simulink model "mat_acc"  (Simulink 8.7)
settings: Solver=VariableStepDiscrete  StartTime=0.0  StopTime=Accelerator_A10_param.endTime  MaxStep=1  RelTol=1e-3
PreLoadFcn:
  | % Run the setup script when the model is opened
  | setup_mat_acc;
InitFcn:
  | % Run the setup script again just before the
  | % model is run, so that any updates made
  | % after opening are applied.
  | setup_mat_acc;
undefined symbols (not defined in the file or in its folder): AdvDSPBChannelOutDisplay, dpoly, dspba_ChannelInVis, dspba_ChannelOutVis, dspba_internal_get_channel_ports, evalAionMaskParam, latency, primtype, value
libraries: DSPBAPrim x1114, DSPBAAvalonST x8, DSPBABase x5, DSPBAControl x2
(part 1 of 5)
Description:
  | DSP Builder Advanced Template for Template Design implementing Primitive Subsystems
settings Model: Creator=mjervis  LastModifiedBy=5g
settings DataIOCC: SignalLoggingSaveFormat=ModelDataLogs
settings OptimizationCC: ExpressionDepthLimit=2147483647
settings DebuggingCC: SolverPrmCheckMsg=warning  InheritedTsInSrcMsg=none  IntegerOverflowMsg=none  FcnCallInpInsideContextMsg=UseLocalSettings  AllowSymbolicDim=off  StateNameClashWarn=warning  IntegerSaturationMsg=none
settings GRTTargetCC: CombineOutputUpdateFcns=off  GRTInterface=on

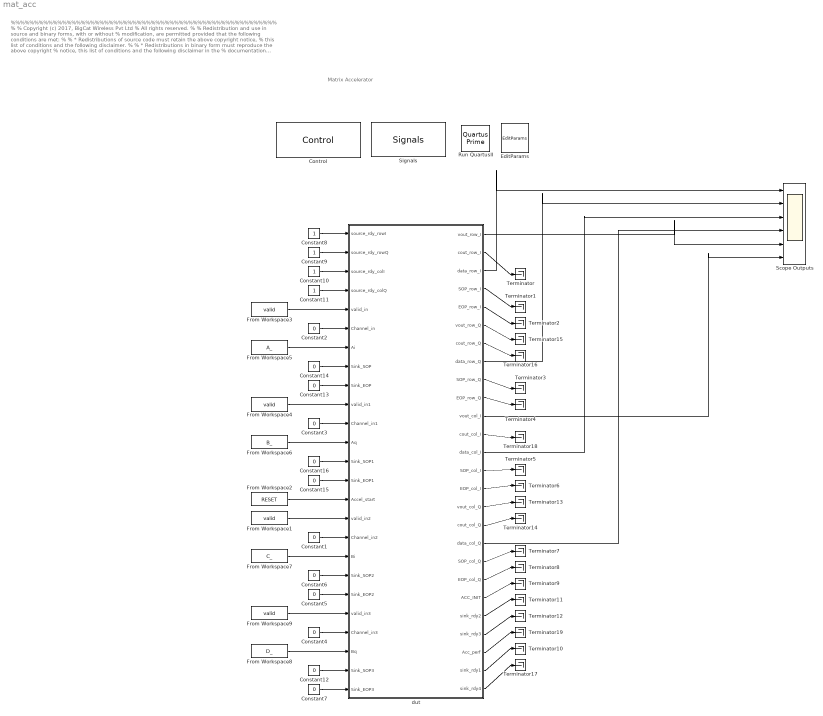
== system mat_acc ==
  note: %%%%%%%%%%%%%%%%%%%%%%%%%%%%%%%%%%%%%%%%%%%%%%%%%%%%%%%%%
      |  %
      |  % Copyright (c) 2017, BigCat Wireless Pvt Ltd
      |  % All rights reserved.
      |  %
      |  % Redistribution and use in source and binary forms, with or without
      |  % modification, are permitted provided that the following conditions are met:
      |  %
      |  %     * Redistributions of source code must retain the above copyright notice,
      |  %       this list of conditions and the following disclaimer.
      |  %
      |  %     * Redistributions in binary form must reproduce the above copyright
      |  %       notice, this list of conditions and the following disclaimer in the
      |  %       documentation and/or other materials provided with the distribution.
      |  %
      |  %     * Neither the name of the copyright holder nor the names of its contributors
      |  %       may be used to endorse or promote products derived from this software
      |  %       without specific prior written permission.
      |  %
      |  %
      |  %
      |  % THIS SOFTWARE IS PROVIDED BY THE COPYRIGHT HOLDERS AND CONTRIBUTORS "AS IS"
      |  % AND ANY EXPRESS OR IMPLIED WARRANTIES, INCLUDING, BUT NOT LIMITED TO, THE
      |  % IMPLIED WARRANTIES OF MERCHANTABILITY AND FITNESS FOR A PARTICULAR PURPOSE ARE
      |  % DISCLAIMED. IN NO EVENT SHALL THE COPYRIGHT HOLDER OR CONTRIBUTORS BE LIABLE
      |  % FOR ANY DIRECT, INDIRECT, INCIDENTAL, SPECIAL, EXEMPLARY, OR CONSEQUENTIAL
      |  % DAMAGES (INCLUDING, BUT NOT LIMITED TO, PROCUREMENT OF SUBSTITUTE GOODS OR
      |  % SERVICES; LOSS OF USE, DATA, OR PROFITS; OR BUSINESS INTERRUPTION) HOWEVER
      |  % CAUSED AND ON ANY THEORY OF LIABILITY, WHETHER IN CONTRACT, STRICT LIABILITY,
      |  % OR TORT (INCLUDING NEGLIGENCE OR OTHERWISE) ARISING IN ANY WAY OUT OF THE USE
      |  % OF THIS SOFTWARE, EVEN IF ADVISED OF THE POSSIBILITY OF SUCH DAMAGE.
      |  %
      |   %%%%%%%%%%%%%%%%%%%%%%%%%%%%%%%%%%%%%%%%%%%%%%%%%%%%%%%%%%
  note: Matrix Accelerator
  Constant{1..4} (4 alike) : Constant  Value=0  OutDataTypeStr=uint8
  Constant{8..11} (4 alike) : Constant  OutDataTypeStr=boolean
  Constant{5..7,12..16} (8 alike) : Constant  Value=0  OutDataTypeStr=boolean
  Control : DSPBABase/Control  generate=on  language=VHDL  destination=./rtl  destination_gui=./rtl  make_full_path=off  path_is_relative=on  autotestbench=on  signaldepth=2  coveragetestbench=off  logs=off  spacewidth=2  spacenum=1  addrwidth=10  datawidth=16  dataendian=Big Endian  hierarchicalnames=off  ramThresholdBits=-1  distRamThresholdBits=-1  mlabThresholdBits=-1  hardMultiplierThresholdLuts=-1  version=20090407  errorOnChanMismatch=1  errorOnGPIOMismatch=0  importModelsimResults=0  cycleAccurate=off  reinterpretCastMult=off  paramFile=mat_acc_params.xml
  EditParams : DSPBABase/EditParams  version=20090407
  From Workspace{1,3..4,9} (4 alike) : FromWorkspace  VariableName=valid  OutDataTypeStr=boolean  SampleTime=0
  From Workspace2 : FromWorkspace  VariableName=RESET  OutDataTypeStr=boolean  SampleTime=0
  From Workspace5 : FromWorkspace  VariableName=A_  SampleTime=0
  From Workspace6 : FromWorkspace  VariableName=B_  SampleTime=0
  From Workspace7 : FromWorkspace  VariableName=C_  SampleTime=0
  From Workspace8 : FromWorkspace  VariableName=D_  SampleTime=0
  "Run QuartusII " : DSPBABase/Quartus Prime  version=20090407
  Scope Outputs : Scope  NumInputPorts=6
  Signals : DSPBABase/Signals  clk=clk  freq=Accelerator_A10_param.ClockRate  margin=Accelerator_A10_param.ClockMargin  rst=areset  rstactive=High  bus=bus  enbusclock=off  busfreq=491.52  bussync=off  version=20090407
  Terminator{,1..19} (20 alike) : Terminator
  dut : Subsystem
  wires:
  Constant8/1 -> dut/1(source_rdy_rowI)
  Constant11/1 -> dut/4(source_rdy_colQ)
  Constant9/1 -> dut/2(source_rdy_rowQ)
  From Workspace2/1 -> dut/15(Accel_start)
  Constant10/1 -> dut/3(source_rdy_colI)
  Constant2/1 -> dut/6(Channel_in)
  Constant3/1 -> dut/11(Channel_in1)
  Constant14/1 -> dut/8(Sink_SOP)
  Constant13/1 -> dut/9(Sink_EOP)
  Constant16/1 -> dut/13(Sink_SOP1)
  Constant15/1 -> dut/14(Sink_EOP1)
  From Workspace3/1 -> dut/5(valid_in)
  From Workspace4/1 -> dut/10(valid_in1)
  dut/3(data_row_I) -> Scope Outputs/1
  dut/8(data_row_Q) -> Scope Outputs/2
  dut/13(data_col_I) -> Scope Outputs/3
  dut/18(data_col_Q) -> Scope Outputs/4
  dut/1(vout_row_I) -> Scope Outputs/5
  dut/11(vout_col_I) -> Scope Outputs/6
  dut/2(cout_row_I) -> Terminator/1
  dut/4(SOP_row_I) -> Terminator1/1
  dut/5(EOP_row_I) -> Terminator2/1
  dut/9(SOP_row_Q) -> Terminator3/1
  dut/10(EOP_row_Q) -> Terminator4/1
  dut/14(SOP_col_I) -> Terminator5/1
  dut/15(EOP_col_I) -> Terminator6/1
  dut/19(SOP_col_Q) -> Terminator7/1
  dut/20(EOP_col_Q) -> Terminator8/1
  dut/21(ACC_INIT) -> Terminator9/1
  dut/22(sink_rdy2) -> Terminator11/1
  dut/23(sink_rdy3) -> Terminator12/1
  dut/16(vout_col_Q) -> Terminator13/1
  dut/17(cout_col_Q) -> Terminator14/1
  dut/6(vout_row_Q) -> Terminator15/1
  dut/7(cout_row_Q) -> Terminator16/1
  dut/12(cout_col_I) -> Terminator18/1
  dut/24(Acc_perf) -> Terminator19/1
  From Workspace5/1 -> dut/7(Ai)
  From Workspace6/1 -> dut/12(Aq)
  From Workspace7/1 -> dut/18(Bi)
  From Workspace8/1 -> dut/23(Bq)
  From Workspace1/1 -> dut/16(valid_in2)
  From Workspace9/1 -> dut/21(valid_in3)
  Constant1/1 -> dut/17(Channel_in2)
  Constant4/1 -> dut/22(Channel_in3)
  Constant6/1 -> dut/19(Sink_SOP2)
  Constant5/1 -> dut/20(Sink_EOP2)
  Constant12/1 -> dut/24(Sink_SOP3)
  Constant7/1 -> dut/25(Sink_EOP3)
  dut/26(sink_rdy4) -> Terminator17/1
  dut/25(sink_rdy1) -> Terminator10/1

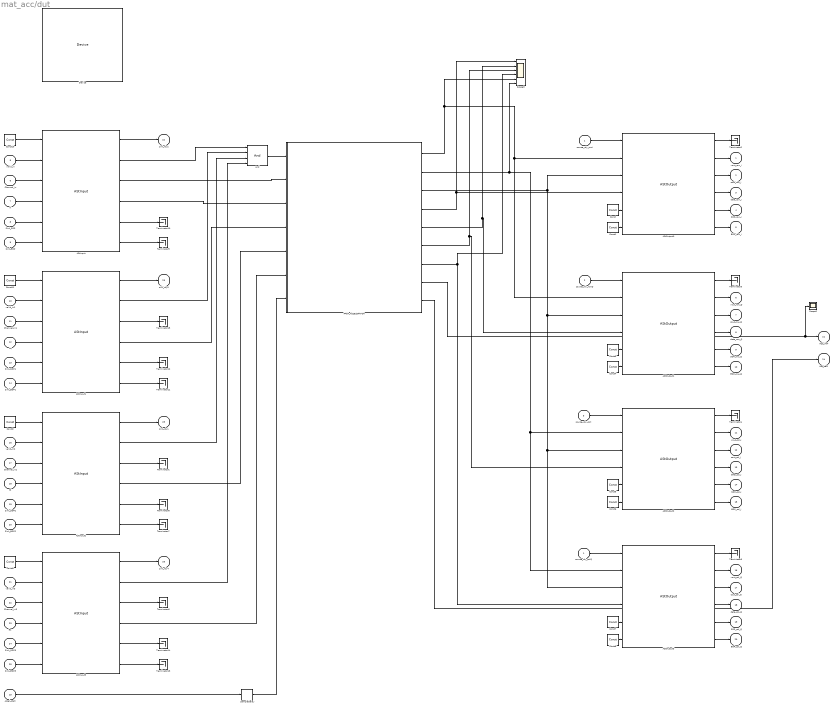
== system mat_acc/dut ==
  source_rdy_rowI : Inport
  source_rdy_rowQ : Inport  Port=2
  source_rdy_colI : Inport  Port=3
  source_rdy_colQ : Inport  Port=4
  valid_in : Inport  Port=5
  Channel_in : Inport  Port=6
  Ai : Inport  Port=7
  Sink_SOP : Inport  Port=8
  Sink_EOP : Inport  Port=9
  valid_in1 : Inport  Port=10
  Channel_in1 : Inport  Port=11
  Aq : Inport  Port=12
  Sink_SOP1 : Inport  Port=13
  Sink_EOP1 : Inport  Port=14
  Accel_start : Inport  Port=15
  valid_in2 : Inport  Port=16
  Channel_in2 : Inport  Port=17
  Bi : Inport  Port=18
  Sink_SOP2 : Inport  Port=19
  Sink_EOP2 : Inport  Port=20
  valid_in3 : Inport  Port=21
  Channel_in3 : Inport  Port=22
  Bq : Inport  Port=23
  Sink_SOP3 : Inport  Port=24
  Sink_EOP3 : Inport  Port=25
  AStInput : DSPBAAvalonST/AStInput
      link override ChannelOut: value=3  packetBeginEnabled=off  latency=0
  AStInput1 : DSPBAAvalonST/AStInput
      link override ChannelOut: value=3  packetBeginEnabled=off  latency=0
  AStInput2 : DSPBAAvalonST/AStInput
      link override ChannelOut: value=3  packetBeginEnabled=off  latency=0
  AStInput3 : DSPBAAvalonST/AStInput
      link override ChannelOut: value=3  packetBeginEnabled=off  latency=0
  AStOutput0 : DSPBAAvalonST/AStOutput  fifo_setup=[32 1 20]
      link override ChannelOut: value=4  packetBeginEnabled=off  latency=0
  AStOutput1 : DSPBAAvalonST/AStOutput  fifo_setup=[32 1 20]
      link override ChannelOut: value=4  packetBeginEnabled=off  latency=0
  AStOutput2 : DSPBAAvalonST/AStOutput  fifo_setup=[32 1 20]
      link override ChannelOut: value=4  packetBeginEnabled=off  latency=0
  AStOutput3 : DSPBAAvalonST/AStOutput  fifo_setup=[32 1 20]
      link override ChannelOut: value=4  packetBeginEnabled=off  latency=0
  And : DSPBAPrim/And  primtype=and  nInputs=4  nOutputs=1  omode=Inherit via internal rule  otype=sfix(16)  scale=2^-15  rndmethod=Unbiased  factor=1  satmethod=Symmetric  shift_vec=[0 1 2 -1]  value=0  inPortNames=[' '; ' '; ' '; ' '; ' '; ' '; ' '; ' '; ' '; ' '; ' '; ' '; ' '; ' '; ' '; ' '; ]  outPortNames=[' ']  dspbaimage=dspba_prim.jpg  text=fprintf('&');  style=Optimised  visibilities=8+2  version=20090407
  Const{,1,3..8} (8 alike) : DSPBAPrim/Const  primtype=const  nInputs=0  nOutputs=1  omode=boolean  otype=sfix(16)  scale=2^-15  rndmethod=Unbiased  factor=1  satmethod=Symmetric  shift_vec=[0 1 2 -1]  value=0  inPortNames=['+'; '+';]  outPortNames=[' ']  dspbaimage=dspba_prim.jpg  text=fprintf('%s', num2str(value));  style=Optimised  visibilities=8 + 1024  floatPrecision=float32_m23  version=20120820
  Const{2,9..11} (4 alike) : DSPBAPrim/Const  primtype=const  nInputs=0  nOutputs=1  omode=boolean  otype=sfix(16)  scale=2^-15  rndmethod=Unbiased  factor=1  satmethod=Symmetric  shift_vec=[0 1 2 -1]  value=1  inPortNames=['+'; '+';]  outPortNames=[' ']  dspbaimage=dspba_prim.jpg  text=fprintf('%s', num2str(value));  style=Optimised  visibilities=8 + 1024  floatPrecision=float32_m23  version=20120820
  Device : DSPBABase/Device  family=Arria 10  deviceMember=Arria 10  stratix4device=Stratix IV E  hardcopy4device=HardCopy IV E  stratix5device=Stratix V GX  device=10AS066N3F40E2SGE2  speed=2  stratixSpeed=-5  stratix2Speed=-3  stratix3Speed=-2  stratix4gxSpeed=-2  stratix4gtSpeed=-1  cyclone2Speed=-6  cyclone3Speed=-7  arria2Speed=-4  cyclone4eSpeed=-8  stratix5Speed=-3  arria5Speed=-4  arriaSpeed=-6  cyclone3lsSpeed=-7  cyclone5Speed=-6  arria2gzSpeed=-3  nightFurySpeed=-2  ecp2Speed=-7  hardcopycompat=off  version=20140217  max10flashmode=off  max10nomeminit=off
  FPGA_ACCELERATOR : Subsystem
  SampleDelay : DSPBAPrim/SampleDelay  primtype=sampdelay  nInputs=1  nOutputs=1  omode=Inherit via internal rule  otype=sfix(16)  scale=2^-15  rndmethod=Unbiased  factor=1  satmethod=Symmetric  shift_vec=[0 1 2 -1]  value=1  inPortNames=[' '; ' ';]  outPortNames=[' ']  dspbaimage=dspba_prim.jpg  text=dpoly(1, eye(1,value+1), 'z')  style=Optimised  visibilities=8 + 1024 + 2^17 + 2^18  flexible=off  slackgroup=0  augmented=0  version=20090407  advOptions=[]
  Scope2 : Scope
  Scope3 : Scope  NumInputPorts=6
  Terminator{1..15} (15 alike) : Terminator
  vout_row_I : Outport
  cout_row_I : Outport  Port=2
  data_row_I : Outport  Port=3
  SOP_row_I : Outport  Port=4
  EOP_row_I : Outport  Port=5
  vout_row_Q : Outport  Port=6
  cout_row_Q : Outport  Port=7
  data_row_Q : Outport  Port=8
  SOP_row_Q : Outport  Port=9
  EOP_row_Q : Outport  Port=10
  vout_col_I : Outport  Port=11
  cout_col_I : Outport  Port=12
  data_col_I : Outport  Port=13
  SOP_col_I : Outport  Port=14
  EOP_col_I : Outport  Port=15
  vout_col_Q : Outport  Port=16
  cout_col_Q : Outport  Port=17
  data_col_Q : Outport  Port=18
  SOP_col_Q : Outport  Port=19
  EOP_col_Q : Outport  Port=20
  ACC_INIT : Outport  Port=21
  sink_rdy2 : Outport  Port=22
  sink_rdy3 : Outport  Port=23
  Acc_perf : Outport  Port=24
  sink_rdy1 : Outport  Port=25
  sink_rdy4 : Outport  Port=26
  wires:
  FPGA_ACCELERATOR/1(R_vout) -> AStOutput0/2, AStOutput1/2, Scope3/5
  FPGA_ACCELERATOR/3(cout) -> AStOutput1/3, AStOutput2/3, AStOutput3/3, AStOutput0/3
  FPGA_ACCELERATOR/4(Row_i) -> Scope3/1, AStOutput0/4
  AStOutput0/2 -> vout_row_I/1
  AStOutput0/3 -> cout_row_I/1
  source_rdy_rowI/1 -> AStOutput0/1
  AStOutput0/1 -> Terminator2/1
  Const/1 -> AStOutput0/5
  Const1/1 -> AStOutput0/6
  AStOutput0/4 -> data_row_I/1
  FPGA_ACCELERATOR/2(Col_vout) -> AStOutput2/2, AStOutput3/2, Scope3/6
  FPGA_ACCELERATOR/5(Row_q) -> Scope3/2, AStOutput1/4
  FPGA_ACCELERATOR/6(Col_i) -> Scope3/3, AStOutput2/4
  FPGA_ACCELERATOR/7(Col_q) -> Scope3/4, AStOutput3/4
  Const3/1 -> AStOutput1/5
  Const4/1 -> AStOutput1/6
  Const5/1 -> AStOutput2/5
  Const6/1 -> AStOutput2/6
  Const7/1 -> AStOutput3/5
  Const8/1 -> AStOutput3/6
  source_rdy_rowQ/1 -> AStOutput1/1
  source_rdy_colI/1 -> AStOutput2/1
  source_rdy_colQ/1 -> AStOutput3/1
  AStOutput3/1 -> Terminator5/1
  AStOutput2/1 -> Terminator4/1
  AStOutput1/1 -> Terminator3/1
  AStOutput1/2 -> vout_row_Q/1
  AStOutput1/3 -> cout_row_Q/1
  AStOutput1/4 -> data_row_Q/1
  AStOutput2/2 -> vout_col_I/1
  AStOutput2/3 -> cout_col_I/1
  AStOutput2/4 -> data_col_I/1
  AStOutput3/2 -> vout_col_Q/1
  AStOutput3/3 -> cout_col_Q/1
  AStOutput3/4 -> data_col_Q/1
  AStOutput0/5 -> SOP_row_I/1
  AStOutput0/6 -> EOP_row_I/1
  AStOutput1/5 -> SOP_row_Q/1
  AStOutput1/6 -> EOP_row_Q/1
  AStOutput3/5 -> SOP_col_Q/1
  AStOutput3/6 -> EOP_col_Q/1
  AStOutput2/5 -> SOP_col_I/1
  AStOutput2/6 -> EOP_col_I/1
  AStInput/5 -> Terminator10/1
  AStInput/6 -> Terminator9/1
  AStInput1/5 -> Terminator12/1
  AStInput1/6 -> Terminator11/1
  Channel_in/1 -> AStInput/3
  valid_in/1 -> AStInput/2
  Ai/1 -> AStInput/4
  Sink_SOP/1 -> AStInput/5
  Sink_EOP/1 -> AStInput/6
  Channel_in1/1 -> AStInput1/3
  valid_in1/1 -> AStInput1/2
  Aq/1 -> AStInput1/4
  Sink_SOP1/1 -> AStInput1/5
  Sink_EOP1/1 -> AStInput1/6
  And/1 -> FPGA_ACCELERATOR/1(Valid_in)
  AStInput/2 -> And/1
  AStInput1/2 -> And/2
  AStInput/1 -> sink_rdy2/1
  AStInput1/1 -> sink_rdy3/1
  AStInput/3 -> FPGA_ACCELERATOR/2(channel_in)
  AStInput1/3 -> Terminator15/1
  SampleDelay/1 -> FPGA_ACCELERATOR/7(Start_of_operation)
  Const10/1 -> AStInput/1
  Const11/1 -> AStInput1/1
  Accel_start/1 -> SampleDelay/1
  FPGA_ACCELERATOR/9(Acc_perf) -> Acc_perf/1
  FPGA_ACCELERATOR/8(Acc_init) -> Scope2/1, ACC_INIT/1
  AStInput/4 -> FPGA_ACCELERATOR/3(Ai)
  AStInput1/4 -> FPGA_ACCELERATOR/4(Aq)
  Channel_in2/1 -> AStInput2/3
  valid_in2/1 -> AStInput2/2
  Bi/1 -> AStInput2/4
  Sink_SOP2/1 -> AStInput2/5
  Sink_EOP2/1 -> AStInput2/6
  Const2/1 -> AStInput2/1
  Channel_in3/1 -> AStInput3/3
  valid_in3/1 -> AStInput3/2
  Bq/1 -> AStInput3/4
  Sink_SOP3/1 -> AStInput3/5
  Sink_EOP3/1 -> AStInput3/6
  Const9/1 -> AStInput3/1
  AStInput2/1 -> sink_rdy1/1
  AStInput3/1 -> sink_rdy4/1
  AStInput2/2 -> And/3
  AStInput3/2 -> And/4
  AStInput2/3 -> Terminator1/1
  AStInput3/3 -> Terminator6/1
  AStInput2/5 -> Terminator8/1
  AStInput2/6 -> Terminator7/1
  AStInput3/5 -> Terminator14/1
  AStInput3/6 -> Terminator13/1
  AStInput2/4 -> FPGA_ACCELERATOR/5(Bi)
  AStInput3/4 -> FPGA_ACCELERATOR/6(Bq)

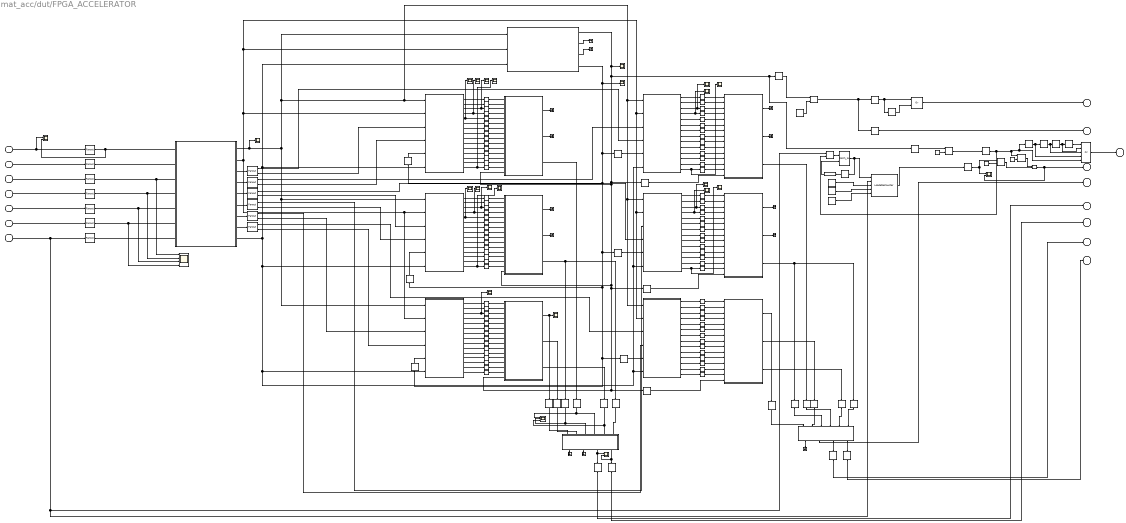
== system mat_acc/dut/FPGA_ACCELERATOR ==
  Valid_in : Inport
  channel_in : Inport  Port=2
  Ai : Inport  Port=3
  Aq : Inport  Port=4
  Bi : Inport  Port=5
  Bq : Inport  Port=6
  Start_of_operation : Inport  Port=7
  12FP_MAC : Subsystem
  12FP_MAC1 : Subsystem
  12FP_MAC2 : Subsystem
  12FP_MUX : Subsystem
  12FP_MUX1 : Subsystem
  12FP_MUX2 : Subsystem
  13FP_MAC : Subsystem
  13FP_MAC1 : Subsystem
  13FP_MAC2 : Subsystem
  13FP_MUX : Subsystem
  13FP_MUX1 : Subsystem
  13FP_MUX2 : Subsystem
  COLUMN_I_and_Q : Subsystem
  CmpEQ : DSPBAPrim/CmpEQ  primtype=cmpeq  nInputs=2  nOutputs=1  omode=boolean  otype=sfix(16)  scale=2^-15  rndmethod=Unbiased  factor=1  satmethod=Symmetric  shift_vec=[0 1 2 -1]  value=0  inPortNames=[' '; ' ';]  outPortNames=[' ']  dspbaimage=dspba_prim.jpg  text=fprintf('==');  style=Optimised  visibilities=0  advOptions=[]  version=20130117
  CmpGE : DSPBAPrim/CmpGE  primtype=cmpgte  nInputs=2  nOutputs=1  omode=boolean  otype=sfix(16)  scale=2^-15  rndmethod=Unbiased  factor=1  satmethod=Symmetric  shift_vec=[0 1 2 -1]  value=0  inPortNames=['a'; 'b';]  outPortNames=[' ']  dspbaimage=dspba_prim.jpg  text=fprintf('a>=b');  style=Optimised  visibilities=0  advOptions=[]  version=20130117
  Const : DSPBAPrim/Const  primtype=const  nInputs=0  nOutputs=1  omode=Inherit via internal rule  otype=sfix(16)  scale=2^-15  rndmethod=Unbiased  factor=1  satmethod=Symmetric  shift_vec=[0 1 2 -1]  value=1  inPortNames=['+'; '+';]  outPortNames=[' ']  dspbaimage=dspba_prim.jpg  text=fprintf('%s', num2str(value));  style=Optimised  visibilities=8 + 1024  floatPrecision=float32_m23  version=20120820
  Const1 : DSPBAPrim/Const  primtype=const  nInputs=0  nOutputs=1  omode=Inherit via internal rule  otype=sfix(16)  scale=2^-15  rndmethod=Unbiased  factor=1  satmethod=Symmetric  shift_vec=[0 1 2 -1]  value=1  inPortNames=['+'; '+';]  outPortNames=[' ']  dspbaimage=dspba_prim.jpg  text=fprintf('%s', num2str(value));  style=Optimised  visibilities=8 + 1024  floatPrecision=float32_m23  version=20120820
  Const2 : DSPBAPrim/Const  primtype=const  nInputs=0  nOutputs=1  omode=Inherit via internal rule  otype=sfix(16)  scale=2^-15  rndmethod=Unbiased  factor=1  satmethod=Symmetric  shift_vec=[0 1 2 -1]  value=0  inPortNames=['+'; '+';]  outPortNames=[' ']  dspbaimage=dspba_prim.jpg  text=fprintf('%s', num2str(value));  style=Optimised  visibilities=8 + 1024  floatPrecision=float32_m23  version=20120820
  Const3 : DSPBAPrim/Const  primtype=const  nInputs=0  nOutputs=1  omode=Inherit via internal rule  otype=sfix(16)  scale=2^-15  rndmethod=Unbiased  factor=1  satmethod=Symmetric  shift_vec=[0 1 2 -1]  value=100000  inPortNames=['+'; '+';]  outPortNames=[' ']  dspbaimage=dspba_prim.jpg  text=fprintf('%s', num2str(value));  style=Optimised  visibilities=8 + 1024  floatPrecision=float32_m23  version=20120820
  Const4 : DSPBAPrim/Const  primtype=const  nInputs=0  nOutputs=1  omode=Inherit via internal rule  otype=sfix(16)  scale=2^-15  rndmethod=Unbiased  factor=1  satmethod=Symmetric  shift_vec=[0 1 2 -1]  value=1  inPortNames=['+'; '+';]  outPortNames=[' ']  dspbaimage=dspba_prim.jpg  text=fprintf('%s', num2str(value));  style=Optimised  visibilities=8 + 1024  floatPrecision=float32_m23  version=20120820
  Const6 : DSPBAPrim/Const  primtype=const  nInputs=0  nOutputs=1  omode=boolean  otype=sfix(16)  scale=2^-15  rndmethod=Unbiased  factor=1  satmethod=Symmetric  shift_vec=[0 1 2 -1]  value=1  inPortNames=['+'; '+';]  outPortNames=[' ']  dspbaimage=dspba_prim.jpg  text=fprintf('%s', num2str(value));  style=Optimised  visibilities=8 + 1024  floatPrecision=float32_m23  version=20120820
  Const7 : DSPBAPrim/Const  primtype=const  nInputs=0  nOutputs=1  omode=Specify via dialog  otype=ufix(1)  scale=2^0  rndmethod=Unbiased  factor=1  satmethod=Symmetric  shift_vec=[0 1 2 -1]  value=1  inPortNames=['+'; '+';]  outPortNames=[' ']  dspbaimage=dspba_prim.jpg  text=fprintf('%s', num2str(value));  style=Optimised  visibilities=8 + 1024  floatPrecision=float32_m23  version=20120820
  Convert : DSPBAPrim/Convert  primtype=convert  nInputs=1  nOutputs=1  omode=boolean  otype=sfix(16)  scale=2^-15  rndmethod=Unbiased  factor=1  satmethod=None  shift_vec=[0 1 2 -1]  value=round([0:255]/17)  inPortNames=[' '; ' ';]  outPortNames=[' '; 'c']  dspbaimage=dspba_prim.jpg  text=fprintf('convert');  style=Optimised  visibilities=8+64+256+2^17  clipdetect=off  floatPrecision=float32_m23  advOptions=[]  version=20130211
  Counter_control_logic : Subsystem
  Fanout{,1..6,13..115} (110 alike) : DSPBAPrim/Fanout  primtype=fanout  nInputs=1  nOutputs=evalAionMaskParam(gcb,'value',1)  omode=Inherit via internal rule  otype=sfix(16)  scale=2^-15  rndmethod=Unbiased  factor=1  satmethod=Symmetric  shift_vec=[0 1 2 -1]  value=1  inPortNames=[' '; ' ';]  outPortNames=[' ']  dspbaimage=dspba_prim.jpg  text=fprintf('fanout')  style=Optimised  visibilities=2^10+2^18  version=20150501  uninit=off
  Fanout{7..12} (6 alike) : DSPBAPrim/Fanout  primtype=fanout  nInputs=1  nOutputs=evalAionMaskParam(gcb,'value',1)  omode=Inherit via internal rule  otype=sfix(16)  scale=2^-15  rndmethod=Unbiased  factor=1  satmethod=Symmetric  shift_vec=[0 1 2 -1]  value=2  inPortNames=[' '; ' ';]  outPortNames=[' ']  dspbaimage=dspba_prim.jpg  text=fprintf('fanout')  style=Optimised  visibilities=2^10+2^18  version=20150501  uninit=off
  Input_operations : Subsystem
  LShift : DSPBAPrim/LShift  primtype=lshift  nInputs=2  nOutputs=1  omode=Specify via dialog  otype=ufix(32)  scale=2^0  rndmethod=Unbiased  factor=1  satmethod=Symmetric  shift_vec=[0 1 2 -1]  value=0  inPortNames=['a'; 'b';]  outPortNames=[' ']  dspbaimage=dspba_prim.jpg  text=fprintf('a << b');  style=Optimised  visibilities=8  version=20090407
  LoadableCounter : DSPBAPrim/LoadableCounter  primtype=loadablecounter  nInputs=5  nOutputs=1  omode=Inherit via internal rule  otype=ufix(16)  scale=2^-0  rndmethod=Unbiased  factor=1  satmethod=Symmetric  shift_vec=[0 1 2 -1]  value=[0 1 0]  inPortNames=['en';'ld';'i ';'s ';'m ']  outPortNames=[' ']  dspbaimage=dspba_prim.jpg  text=fprintf('loadable\ncounter\n[%d %d %d]', value(1), value(2), value(3));  style=Optimised  visibilities=8 + 1024  version=20090407
  Not1 : DSPBAPrim/Not  primtype=not  nInputs=1  nOutputs=1  omode=Inherit via internal rule  otype=sfix(16)  scale=2^-15  rndmethod=Unbiased  factor=1  satmethod=Symmetric  shift_vec=[0 1 2 -1]  value=0  inPortNames=[' '; ' ';]  outPortNames=[' ']  dspbaimage=dspba_prim.jpg  text=fprintf('~');  style=Optimised  visibilities=8  version=20090407
  Or : DSPBAPrim/Or  primtype=or  nInputs=2  nOutputs=1  omode=Inherit via internal rule  otype=sfix(16)  scale=2^-15  rndmethod=Unbiased  factor=1  satmethod=Symmetric  shift_vec=[0 1 2 -1]  value=0  inPortNames=[' '; ' '; ' '; ' '; ' '; ' '; ' '; ' '; ' '; ' '; ' '; ' '; ' '; ' '; ' '; ' '; ]  outPortNames=[' ']  dspbaimage=dspba_prim.jpg  text=fprintf('|');  style=Optimised  visibilities=8+2  version=20090407
  Or1 : DSPBAPrim/Or  primtype=or  nInputs=2  nOutputs=1  omode=Inherit via internal rule  otype=sfix(16)  scale=2^-15  rndmethod=Unbiased  factor=1  satmethod=Symmetric  shift_vec=[0 1 2 -1]  value=0  inPortNames=[' '; ' '; ' '; ' '; ' '; ' '; ' '; ' '; ' '; ' '; ' '; ' '; ' '; ' '; ' '; ' '; ]  outPortNames=[' ']  dspbaimage=dspba_prim.jpg  text=fprintf('|');  style=Optimised  visibilities=8+2  version=20090407
  Or2 : DSPBAPrim/Or  primtype=or  nInputs=2  nOutputs=1  omode=Inherit via internal rule  otype=sfix(16)  scale=2^-15  rndmethod=Unbiased  factor=1  satmethod=Symmetric  shift_vec=[0 1 2 -1]  value=0  inPortNames=[' '; ' '; ' '; ' '; ' '; ' '; ' '; ' '; ' '; ' '; ' '; ' '; ' '; ' '; ' '; ' '; ]  outPortNames=[' ']  dspbaimage=dspba_prim.jpg  text=fprintf('|');  style=Optimised  visibilities=8+2  version=20090407
  Or3 : DSPBAPrim/Or  primtype=or  nInputs=5  nOutputs=1  omode=Inherit via internal rule  otype=sfix(16)  scale=2^-15  rndmethod=Unbiased  factor=1  satmethod=Symmetric  shift_vec=[0 1 2 -1]  value=0  inPortNames=[' '; ' '; ' '; ' '; ' '; ' '; ' '; ' '; ' '; ' '; ' '; ' '; ' '; ' '; ' '; ' '; ]  outPortNames=[' ']  dspbaimage=dspba_prim.jpg  text=fprintf('|');  style=Optimised  visibilities=8+2  version=20090407
  ROW_I_and_Q : Subsystem
  SampleDelay{3..5,93,95..96,98..99,105..108,110..115} (18 alike) : DSPBAPrim/SampleDelay  primtype=sampdelay  nInputs=1  nOutputs=1  omode=Inherit via internal rule  otype=sfix(16)  scale=2^-15  rndmethod=Unbiased  factor=1  satmethod=Symmetric  shift_vec=[0 1 2 -1]  value=1  inPortNames=[' '; ' ';]  outPortNames=[' ']  dspbaimage=dspba_prim.jpg  text=dpoly(1, eye(1,value+1), 'z')  style=Optimised  visibilities=8 + 1024 + 2^17 + 2^18  flexible=off  slackgroup=0  augmented=0  version=20090407  advOptions=[]
  SampleDelay109 : DSPBAPrim/SampleDelay  primtype=sampdelay  nInputs=1  nOutputs=1  omode=Inherit via internal rule  otype=sfix(16)  scale=2^-15  rndmethod=Unbiased  factor=1  satmethod=Symmetric  shift_vec=[0 1 2 -1]  value=8  inPortNames=[' '; ' ';]  outPortNames=[' ']  dspbaimage=dspba_prim.jpg  text=dpoly(1, eye(1,value+1), 'z')  style=Optimised  visibilities=8 + 1024 + 2^17 + 2^18  flexible=off  slackgroup=0  augmented=0  version=20090407  advOptions=[]
  SampleDelay94 : DSPBAPrim/SampleDelay  primtype=sampdelay  nInputs=1  nOutputs=1  omode=Inherit via internal rule  otype=sfix(16)  scale=2^-15  rndmethod=Unbiased  factor=1  satmethod=Symmetric  shift_vec=[0 1 2 -1]  value=11  inPortNames=[' '; ' ';]  outPortNames=[' ']  dspbaimage=dspba_prim.jpg  text=dpoly(1, eye(1,value+1), 'z')  style=Optimised  visibilities=8 + 1024 + 2^17 + 2^18  flexible=off  slackgroup=0  augmented=0  version=20090407  advOptions=[]
  Scope{,2,4..6,8..18,20..22} (19 alike) : Scope
  Scope1 : Scope  NumInputPorts=2
  Scope19 : Scope  NumInputPorts=2
  Scope23 : Scope  NumInputPorts=2
  Scope3 : Scope  NumInputPorts=3
  Scope7 : Scope  NumInputPorts=4
  Terminator{,1..4,7..9,11..15} (13 alike) : Terminator
  latch_1L : DSPBAControl/latch_1L
  latch_1L1 : DSPBAControl/latch_1L
  R_vout : Outport
  Col_vout : Outport  Port=2
  cout : Outport  Port=3
  Row_i : Outport  Port=4
  Row_q : Outport  Port=5
  Col_i : Outport  Port=6
  Col_q : Outport  Port=7
  Acc_init : Outport  Port=8
  Acc_perf : Outport  Port=9
  wires:
  Counter_control_logic/1(Count) -> SampleDelay4/1, 13FP_MUX2/16(MUX_select), SampleDelay5/1, 13FP_MUX1/16(MUX_select), 13FP_MUX/16(MUX_select), SampleDelay3/1, SampleDelay109/1, SampleDelay94/1, Scope/1
  Fanout9/1 -> 12FP_MAC1/4(Ai-Aq)
  13FP_MUX1/3((Ai-Aq)*Bq) -> Fanout104/1, Fanout102/1
  12FP_MUX2/3((Bi+Bq)*Aq) -> Fanout110/1
  13FP_MUX2/3(Aq*(Bi+Bq)) -> Fanout105/1
  12FP_MAC1/4(M1) -> Fanout75/1, Scope18/1
  12FP_MAC2/12(M9) -> Fanout97/1
  12FP_MAC1/12(M9) -> Fanout83/1
  12FP_MAC2/4(M1) -> Fanout89/1
  12FP_MAC2/7(M4) -> Fanout92/1
  12FP_MAC2/9(M6) -> Fanout94/1
  12FP_MAC1/3(M0) -> Fanout74/1, Scope6/1
  12FP_MAC2/1(vout) -> Fanout86/1
  12FP_MAC2/3(M0) -> Fanout88/1
  12FP_MUX/3((Bi-Bq)*Ai) -> Fanout109/1
  12FP_MAC/4(M1) -> Fanout61/1, Scope17/1
  12FP_MAC/6(M3) -> Fanout63/1
  12FP_MAC/10(M7) -> Fanout67/1
  12FP_MAC2/14(M11) -> Fanout99/1
  12FP_MAC1/13(M10) -> Fanout84/1
  12FP_MAC1/6(M3) -> Fanout77/1
  12FP_MAC1/7(M4) -> Fanout78/1
  12FP_MUX1/3(Bq*(Ai-Aq)) -> Fanout111/1, Fanout108/1
  12FP_MAC/13(M10) -> Fanout70/1
  12FP_MAC1/8(M5) -> Fanout79/1
  12FP_MAC2/8(M5) -> Fanout93/1
  12FP_MAC2/13(M10) -> Fanout98/1
  12FP_MAC2/11(M8) -> Fanout96/1
  12FP_MAC1/9(M6) -> Fanout80/1
  12FP_MAC1/2(cout) -> Fanout73/1
  12FP_MAC1/11(M8) -> Fanout82/1
  12FP_MAC1/10(M7) -> Fanout81/1
  12FP_MAC2/10(M7) -> Fanout95/1
  12FP_MAC2/5(M2) -> Fanout90/1
  12FP_MAC1/14(M11) -> Fanout85/1, Scope15/1
  12FP_MAC/11(M8) -> Fanout68/1
  12FP_MAC2/2(cout) -> Fanout87/1
  12FP_MAC/9(M6) -> Fanout66/1
  13FP_MAC1/6(M3) -> Fanout33/1
  13FP_MAC/4(M1) -> Fanout16/1, Scope9/1
  13FP_MAC2/10(M7) -> Fanout52/1
  13FP_MAC1/4(M1) -> Fanout31/1, Scope10/1
  13FP_MAC/9(M6) -> Fanout21/1
  12FP_MAC/8(M5) -> Fanout65/1
  13FP_MAC1/5(M2) -> Fanout32/1, Scope12/1
  12FP_MAC2/6(M3) -> Fanout91/1
  13FP_MAC/5(M2) -> Fanout17/1, Scope11/1
  13FP_MAC/11(M8) -> Fanout23/1
  13FP_MAC2/2(cout) -> Fanout44/1
  13FP_MUX/3(Ai*(Bi-Bq)) -> Fanout103/1
  12FP_MAC1/5(M2) -> Fanout76/1
  13FP_MAC2/11(M8) -> Fanout53/1
  13FP_MAC1/9(M6) -> Fanout36/1
  13FP_MAC/7(M4) -> Fanout19/1
  12FP_MAC/12(M9) -> Fanout69/1
  13FP_MAC/14(M11) -> Fanout26/1
  13FP_MAC2/8(M5) -> Fanout50/1
  13FP_MAC/10(M7) -> Fanout22/1
  13FP_MAC2/3(M0) -> Fanout45/1, Scope8/1
  13FP_MAC2/14(M11) -> Fanout56/1
  12FP_MAC/14(M11) -> Fanout71/1, Scope16/1
  13FP_MAC/3(M0) -> Fanout15/1, Scope2/1
  13FP_MAC2/7(M4) -> Fanout49/1
  13FP_MAC1/8(M5) -> Fanout35/1
  13FP_MAC/2(cout) -> Fanout14/1
  13FP_MAC2/12(M9) -> Fanout54/1
  13FP_MAC/12(M9) -> Fanout24/1
  12FP_MAC/7(M4) -> Fanout64/1
  13FP_MAC1/13(M10) -> Fanout40/1
  12FP_MAC/5(M2) -> Fanout62/1
  13FP_MAC/8(M5) -> Fanout20/1
  13FP_MAC/6(M3) -> Fanout18/1
  13FP_MAC1/10(M7) -> Fanout37/1
  12FP_MAC/1(vout) -> Fanout58/1
  12FP_MAC/2(cout) -> Fanout59/1
  13FP_MAC2/4(M1) -> Fanout46/1
  13FP_MAC1/15(M12) -> Fanout42/1, Scope14/1
  12FP_MAC1/1(vout) -> Fanout72/1
  13FP_MAC1/3(M0) -> Fanout30/1, Scope4/1
  13FP_MAC2/5(M2) -> Fanout47/1
  12FP_MAC/3(M0) -> Fanout60/1, Scope5/1
  13FP_MAC1/7(M4) -> Fanout34/1
  13FP_MAC2/6(M3) -> Fanout48/1
  13FP_MAC2/15(M12) -> Fanout57/1
  13FP_MAC/15(M12) -> Fanout27/1, Scope13/1
  13FP_MAC2/13(M10) -> Fanout55/1
  13FP_MAC2/9(M6) -> Fanout51/1
  13FP_MAC1/11(M8) -> Fanout38/1
  13FP_MAC/1(vout) -> Fanout13/1
  13FP_MAC1/14(M11) -> Fanout41/1
  13FP_MAC1/12(M9) -> Fanout39/1
  13FP_MAC/13(M10) -> Fanout25/1
  SampleDelay3/1 -> 12FP_MUX/15(MUX_select)
  SampleDelay4/1 -> 12FP_MUX1/15(MUX_select)
  SampleDelay5/1 -> 12FP_MUX2/15(MUX_select)
  12FP_MUX/2(cout) -> Terminator/1
  12FP_MUX1/1(vout) -> Terminator1/1
  12FP_MUX1/2(cout) -> Terminator2/1
  12FP_MUX2/1(vout) -> Fanout106/1
  12FP_MUX2/2(cout) -> Fanout107/1
  13FP_MUX2/2(cout) -> Fanout101/1
  13FP_MUX2/1(vout) -> Scope20/1, Fanout100/1
  13FP_MUX1/2(cout) -> Terminator7/1
  13FP_MUX1/1(vout) -> Terminator8/1
  13FP_MUX/2(cout) -> Terminator9/1
  Counter_control_logic/2("Channel out ") -> Terminator11/1
  Counter_control_logic/3(Valid out) -> Terminator12/1
  Fanout103/1 -> ROW_I_and_Q/4(I2), Scope3/1
  Fanout102/1 -> ROW_I_and_Q/3(I1), Scope3/2
  Fanout15/1 -> 13FP_MUX/3(I0)
  Fanout16/1 -> 13FP_MUX/4(I1)
  Fanout17/1 -> 13FP_MUX/5(I2)
  Fanout18/1 -> 13FP_MUX/6(I3)
  Fanout19/1 -> 13FP_MUX/7(I4)
  Fanout20/1 -> 13FP_MUX/8(I5)
  Fanout21/1 -> 13FP_MUX/9(I6)
  Fanout22/1 -> 13FP_MUX/10(I7)
  Fanout23/1 -> 13FP_MUX/11(I8)
  Fanout24/1 -> 13FP_MUX/12(I9)
  Fanout25/1 -> 13FP_MUX/13(I10)
  Fanout26/1 -> 13FP_MUX/14(I11)
  Fanout27/1 -> 13FP_MUX/15(I12)
  13FP_MAC1/1(vout) -> Fanout28/1
  13FP_MAC1/2(cout) -> Fanout29/1
  Fanout30/1 -> 13FP_MUX1/3(I0)
  Fanout31/1 -> 13FP_MUX1/4(I1)
  Fanout32/1 -> 13FP_MUX1/5(I2)
  Fanout33/1 -> 13FP_MUX1/6(I3)
  Fanout34/1 -> 13FP_MUX1/7(I4)
  Fanout35/1 -> 13FP_MUX1/8(I5)
  Fanout36/1 -> 13FP_MUX1/9(I6)
  Fanout37/1 -> 13FP_MUX1/10(I7)
  Fanout38/1 -> 13FP_MUX1/11(I8)
  Fanout39/1 -> 13FP_MUX1/12(I9)
  Fanout40/1 -> 13FP_MUX1/13(I10)
  Fanout41/1 -> 13FP_MUX1/14(I11)
  Fanout42/1 -> 13FP_MUX1/15(I12)
  13FP_MAC2/1(vout) -> Fanout43/1
  Fanout45/1 -> 13FP_MUX2/3(I0)
  Fanout46/1 -> 13FP_MUX2/4(I1)
  Fanout47/1 -> 13FP_MUX2/5(I2)
  Fanout48/1 -> 13FP_MUX2/6(I3)
  Fanout49/1 -> 13FP_MUX2/7(I4)
  Fanout50/1 -> 13FP_MUX2/8(I5)
  Fanout51/1 -> 13FP_MUX2/9(I6)
  Fanout52/1 -> 13FP_MUX2/10(I7)
  Fanout53/1 -> 13FP_MUX2/11(I8)
  Fanout54/1 -> 13FP_MUX2/12(I9)
  Fanout55/1 -> 13FP_MUX2/13(I10)
  Fanout56/1 -> 13FP_MUX2/14(I11)
  Fanout57/1 -> 13FP_MUX2/15(I12)
  Fanout61/1 -> 12FP_MUX/4(I1)
  Fanout62/1 -> 12FP_MUX/5(I2)
  Fanout63/1 -> 12FP_MUX/6(I3)
  Fanout64/1 -> 12FP_MUX/7(I4)
  Fanout65/1 -> 12FP_MUX/8(I5)
  Fanout66/1 -> 12FP_MUX/9(I6)
  Fanout67/1 -> 12FP_MUX/10(I7)
  Fanout68/1 -> 12FP_MUX/11(I8)
  Fanout69/1 -> 12FP_MUX/12(I9)
  Fanout70/1 -> 12FP_MUX/13(I10)
  Fanout71/1 -> 12FP_MUX/14(I11)
  Fanout74/1 -> 12FP_MUX1/3(I0)
  Fanout75/1 -> 12FP_MUX1/4(I1)
  Fanout76/1 -> 12FP_MUX1/5(I2)
  Fanout77/1 -> 12FP_MUX1/6(I3)
  Fanout60/1 -> 12FP_MUX/3(I0)
  Fanout78/1 -> 12FP_MUX1/7(I4)
  Fanout79/1 -> 12FP_MUX1/8(I5)
  Fanout80/1 -> 12FP_MUX1/9(I6)
  Fanout81/1 -> 12FP_MUX1/10(I7)
  Fanout82/1 -> 12FP_MUX1/11(I8)
  Fanout83/1 -> 12FP_MUX1/12(I9)
  Fanout84/1 -> 12FP_MUX1/13(I10)
  Fanout85/1 -> 12FP_MUX1/14(I11)
  Fanout88/1 -> 12FP_MUX2/3(I0)
  Fanout89/1 -> 12FP_MUX2/4(I1)
  Fanout90/1 -> 12FP_MUX2/5(I2)
  Fanout91/1 -> 12FP_MUX2/6(I3)
  Fanout92/1 -> 12FP_MUX2/7(I4)
  Fanout93/1 -> 12FP_MUX2/8(I5)
  Fanout94/1 -> 12FP_MUX2/9(I6)
  Fanout95/1 -> 12FP_MUX2/10(I7)
  Fanout96/1 -> 12FP_MUX2/11(I8)
  Fanout97/1 -> 12FP_MUX2/12(I9)
  Fanout98/1 -> 12FP_MUX2/13(I10)
  Fanout99/1 -> 12FP_MUX2/14(I11)
  SampleDelay93/1 -> Col_vout/1
  Const/1 -> CmpGE/2
  SampleDelay94/1 -> CmpGE/1
  13FP_MUX/1(vout) -> Terminator13/1
  COLUMN_I_and_Q/2(chan_out) -> cout/1
  Fanout12/1 -> 12FP_MAC2/3(Bi+Bq)
  Fanout10/1 -> 12FP_MAC1/3(Bq)
  Fanout11/1 -> 12FP_MAC2/4(Aq)
  channel_in/1 -> Fanout1/1
  Ai/1 -> Fanout2/1
  ROW_I_and_Q/4(Q_ROW) -> Fanout113/1, Scope1/2
  ROW_I_and_Q/3(I_ROW) -> Fanout112/1, Scope1/1
  ROW_I_and_Q/1(Val_out) -> Terminator14/1
  ROW_I_and_Q/2(chan_out) -> Terminator15/1
  Fanout105/1 -> Scope3/3, ROW_I_and_Q/5(Q1)
  Fanout104/1 -> ROW_I_and_Q/6(Q2)
  Fanout110/1 -> COLUMN_I_and_Q/5(Q1)
  Fanout111/1 -> COLUMN_I_and_Q/6(Q2)
  Fanout108/1 -> COLUMN_I_and_Q/3(I1)
  Fanout109/1 -> COLUMN_I_and_Q/4(I2)
  COLUMN_I_and_Q/4(Q_COLUMN) -> Fanout115/1
  COLUMN_I_and_Q/3(I_COLUMN) -> Fanout114/1
  12FP_MUX/1(vout) -> Terminator3/1
  COLUMN_I_and_Q/1(Val_out) -> Terminator4/1
  CmpEQ/1 -> SampleDelay95/1
  Const1/1 -> CmpEQ/2
  SampleDelay95/1 -> latch_1L1/1, Or3/5, SampleDelay105/1, Or/2
  CmpGE/1 -> SampleDelay96/1, SampleDelay93/1
  SampleDelay96/1 -> SampleDelay99/1, Or2/1
  Fanout7/1 -> 12FP_MAC/4(Ai)
  Fanout8/1 -> 12FP_MAC/3(Bi-Bq)
  Input_operations/1(vout) -> Scope21/1, 12FP_MAC2/1(valid), 12FP_MAC1/1(valid), 12FP_MAC/1(valid), 13FP_MAC/1(valid), Counter_control_logic/1(Valid in), 13FP_MAC2/1(valid), 13FP_MAC1/1(valid)
  Input_operations/2(cout) -> 12FP_MAC2/2(channel), 12FP_MAC1/2(channel), 12FP_MAC/2(channel), Counter_control_logic/2(Channel in), 13FP_MAC/2(channel), 13FP_MAC2/2(channel), 13FP_MAC1/2(channel)
  Counter_control_logic/4(Acc_clear) -> SampleDelay111/1, SampleDelay114/1, SampleDelay110/1, SampleDelay115/1, SampleDelay112/1, SampleDelay113/1, Scope22/1
  latch_1L/1 -> Not1/1, LoadableCounter/1
  Const2/1 -> LoadableCounter/3
  Valid_in/1 -> Fanout/1, Scope19/1  "qv"
  Const3/1 -> LoadableCounter/5
  Const4/1 -> LoadableCounter/4
  Or/1 -> latch_1L/1
  Not1/1 -> Convert/1
  LoadableCounter/1 -> SampleDelay98/1
  Convert/1 -> latch_1L/2
  SampleDelay98/1 -> LShift/1, Scope23/1
  Const6/1 -> LShift/2
  LShift/1 -> Or1/2
  latch_1L1/1 -> Or1/1
  Const7/1 -> latch_1L1/2
  SampleDelay99/1 -> Or2/2
  Or2/1 -> R_vout/1
  Input_operations/9(SOP_out) -> Counter_control_logic/3(Load_counter), 13FP_MAC/6(SOP_in), 13FP_MAC2/6(SOP_in), 12FP_MAC2/6(SOP_in), 12FP_MAC/6(SOP_in), 12FP_MAC1/6(SOP_in), 13FP_MAC1/6(SOP_in)
  Aq/1 -> Fanout3/1
  Bi/1 -> Fanout4/1
  Bq/1 -> Fanout5/1
  Fanout/1 -> Scope19/2, Input_operations/1(Valid_in)
  Fanout1/1 -> Input_operations/2(Channel_in)
  Fanout2/1 -> Scope7/1, Input_operations/3(Ai)
  Fanout3/1 -> Scope7/2, Input_operations/4(Aq)
  Fanout4/1 -> Scope7/3, Input_operations/5(Bi)
  Fanout5/1 -> Scope7/4, Input_operations/6(Bq)
  Fanout6/1 -> Input_operations/7(SOP_in)
  SampleDelay105/1 -> Or3/4, SampleDelay107/1
  SampleDelay107/1 -> Or3/3, SampleDelay106/1
  SampleDelay106/1 -> Or3/2, SampleDelay108/1
  SampleDelay108/1 -> Or3/1
  SampleDelay109/1 -> CmpEQ/1
  SampleDelay111/1 -> 13FP_MAC/5(Acc_clear)
  SampleDelay110/1 -> 13FP_MAC1/5(Acc_clear)
  SampleDelay112/1 -> 13FP_MAC2/5(Acc_clear)
  SampleDelay113/1 -> 12FP_MAC/5(Acc_clear)
  SampleDelay114/1 -> 12FP_MAC1/5(Acc_clear)
  SampleDelay115/1 -> 12FP_MAC2/5(Acc_clear)
  Start_of_operation/1 -> Fanout6/1, Or/1, LoadableCounter/2
  Or3/1 -> Acc_init/1
  Or1/1 -> Acc_perf/1, Scope23/2
  Input_operations/3(A_i) -> Fanout7/1
  Input_operations/4(Bi_-_Bq) -> Fanout8/1
  Input_operations/5(Ai_-_Aq) -> Fanout9/1
  Input_operations/6(B_q) -> Fanout10/1
  Input_operations/7(A_q) -> Fanout11/1
  Input_operations/8(Bi_+_Bq) -> Fanout12/1
  Fanout7/2 -> 13FP_MAC/3(Ai)
  Fanout8/2 -> 13FP_MAC/4(Bi-Bq)
  Fanout9/2 -> 13FP_MAC1/3(Ai-Aq)
  Fanout10/2 -> 13FP_MAC1/4(Bq)
  Fanout11/2 -> 13FP_MAC2/3(Aq)
  Fanout12/2 -> 13FP_MAC2/4(Bi+Bq)
  Fanout13/1 -> 13FP_MUX/1(Valid)
  Fanout14/1 -> 13FP_MUX/2(Channel)
  Fanout28/1 -> 13FP_MUX1/1(Valid)
  Fanout29/1 -> 13FP_MUX1/2(Channel)
  Fanout43/1 -> 13FP_MUX2/1(Valid)
  Fanout44/1 -> 13FP_MUX2/2(Channel)
  Fanout58/1 -> 12FP_MUX/1(Valid)
  Fanout59/1 -> 12FP_MUX/2(Channel)
  Fanout72/1 -> 12FP_MUX1/1(Valid)
  Fanout73/1 -> 12FP_MUX1/2(Channel)
  Fanout86/1 -> 12FP_MUX2/1(Valid)
  Fanout87/1 -> 12FP_MUX2/2(Channel)
  Fanout100/1 -> ROW_I_and_Q/1(Val_in)
  Fanout101/1 -> ROW_I_and_Q/2(Chan_in)
  Fanout106/1 -> COLUMN_I_and_Q/1(Val_in)
  Fanout107/1 -> COLUMN_I_and_Q/2(Chan_in)
  Fanout112/1 -> Row_i/1
  Fanout113/1 -> Row_q/1
  Fanout114/1 -> Col_i/1
  Fanout115/1 -> Col_q/1

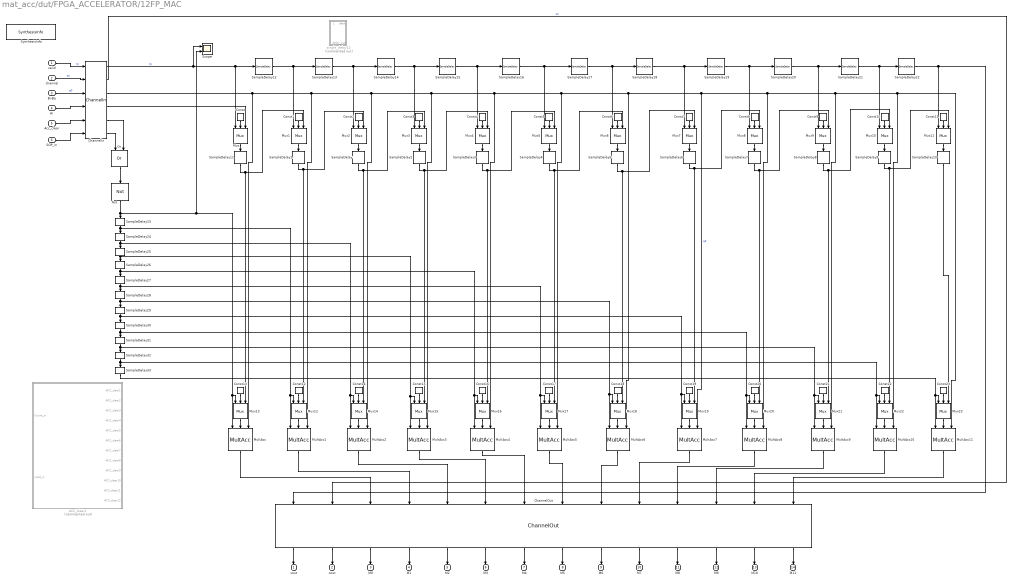
== system mat_acc/dut/FPGA_ACCELERATOR/12FP_MAC ==
  valid : Inport
  channel : Inport  Port=2
  Bi-Bq : Inport  Port=3
  Ai : Inport  Port=4
  Acc_clear : Inport  Port=5
  SOP_in : Inport  Port=6
  ACC_clear1 : Subsystem  Commented=on
  ChannelIn : DSPBAPrim/ChannelIn  primtype=channelin  nInputs=dspba_internal_get_channel_ports(gcb)  nOutputs=dspba_internal_get_channel_ports(gcb)  omode=Inherit via internal rule  otype=sfix(16)  scale=2^-15  rndmethod=Unbiased  factor=1  satmethod=Symmetric  shift_vec=[0 1 2 -1]  value=4  inPortNames=['v'; 'c'; '0'; '1'; '2'; '3'; '4'; '5'; '6'; '7'; '8'; '9'; 'A'; 'B'; 'D'; 'E'; 'F'; 'G'; 'H'; 'I'; 'J'; 'K'; 'L'; 'M'; 'N'; 'O'; 'P'; 'Q'; 'R'; 'S'; 'T'; 'U'; 'W'; 'X'; 'Y'; 'Z']  outPortNames=['v'; 'c'; '0'; '1'; '2'; '3'; '4'; '5'; '6'; '7'; '8'; '9'; 'A'; 'B'; 'D'; 'E'; 'F'; 'G'; 'H'; 'I'; 'J'; 'K'; 'L'; 'M'; 'N'; 'O'; 'P'; 'Q'; 'R'; 'S'; 'T'; 'U'; 'W'; 'X'; 'Y'; 'Z']  dspbaimage=dspba_prim.jpg  text=fprintf('In');  style=Optimised  dataSignals=4  foldingEnabled=off  channels=1  sampleRate=200  packetBeginPresent=off  packetBeginEnabled=off  visibilities=dspba_ChannelInVis(gcb)  latencyCorrection=0  version=20141013
  ChannelOut : DSPBAPrim/ChannelOut  primtype=channelout  nInputs=dspba_internal_get_channel_ports(gcb)  nOutputs=dspba_internal_get_channel_ports(gcb)  omode=Inherit via internal rule  otype=sfix(16)  scale=2^-15  rndmethod=Unbiased  factor=1  satmethod=Symmetric  shift_vec=[0 1 2 -1]  value=12  inPortNames=['v'; 'c'; '0'; '1'; '2'; '3'; '4'; '5'; '6'; '7'; '8'; '9'; 'A'; 'B'; 'D'; 'E'; 'F'; 'G'; 'H'; 'I'; 'J'; 'K'; 'L'; 'M'; 'N'; 'O'; 'P'; 'Q'; 'R'; 'S'; 'T'; 'U'; 'W'; 'X'; 'Y'; 'Z']  outPortNames=['v'; 'c'; '0'; '1'; '2'; '3'; '4'; '5'; '6'; '7'; '8'; '9'; 'A'; 'B'; 'D'; 'E'; 'F'; 'G'; 'H'; 'I'; 'J'; 'K'; 'L'; 'M'; 'N'; 'O'; 'P'; 'Q'; 'R'; 'S'; 'T'; 'U'; 'W'; 'X'; 'Y'; 'Z']  dspbaimage=dspba_prim.jpg  text=fprintf('Out%s', AdvDSPBChannelOutDisplay(latency));  style=Optimised  dataSignals=12  foldingEnabled=off  channels=1  sampleRate=200  packetBeginPresent=off  packetBeginEnabled=off  visibilities=dspba_ChannelOutVis(gcb)  latency=7  latencyCorrection=0  version=20141013
  Const{,1..23} (24 alike) : DSPBAPrim/Const  primtype=const  nInputs=0  nOutputs=1  omode=single  otype=sfix(16)  scale=2^-15  rndmethod=Unbiased  factor=1  satmethod=Symmetric  shift_vec=[0 1 2 -1]  value=0  inPortNames=['+'; '+';]  outPortNames=[' ']  dspbaimage=dspba_prim.jpg  text=fprintf('%s', num2str(value));  style=Optimised  visibilities=8 + 1024  floatPrecision=float32_m23  version=20120820
  MultAcc{,1..11} (12 alike) : DSPBAPrim/MultAcc  primtype=multaccfunc  nInputs=3  nOutputs=1  omode=Inherit via internal rule  otype=sfix(16)  scale=2^-15  rndmethod=Unbiased  factor=1  satmethod=Symmetric  shift_vec=[0 1 2 -1]  value=0  inPortNames="[ 'acc'; 'x  '; 'y  ']"  outPortNames=[]  dspbaimage=dspba_prim_float.jpg  text=disp('multAcc');  style=Optimised  visibilities=8+2^17  functionExpr=fpMultAcc  advOptions=[]  version=20121130
  Mux{,1..23} (24 alike) : DSPBAPrim/Mux  primtype=mux  nInputs=evalAionMaskParam(gcb,'value',1)+1  nOutputs=1  omode=Inherit via internal rule  otype=sfix(16)  scale=2^-15  rndmethod=Unbiased  factor=1  satmethod=Symmetric  shift_vec=[0 1 2 -1]  value=2  inPortNames=['s '; 'd0'; 'd1'; 'd2'; 'd3'; 'd4'; 'd5'; 'd6'; 'd7'; 'd8'; 'd9';]  outPortNames=[' ']  dspbaimage=dspba_prim.jpg  text=fprintf('%s', primtype);  style=Optimised  visibilities=1032  version=20131025
  Not : DSPBAPrim/Not  primtype=not  nInputs=1  nOutputs=1  omode=Inherit via internal rule  otype=sfix(16)  scale=2^-15  rndmethod=Unbiased  factor=1  satmethod=Symmetric  shift_vec=[0 1 2 -1]  value=0  inPortNames=[' '; ' ';]  outPortNames=[' ']  dspbaimage=dspba_prim.jpg  text=fprintf('~');  style=Optimised  visibilities=8  version=20090407
  Or : DSPBAPrim/Or  primtype=or  nInputs=2  nOutputs=1  omode=Inherit via internal rule  otype=sfix(16)  scale=2^-15  rndmethod=Unbiased  factor=1  satmethod=Symmetric  shift_vec=[0 1 2 -1]  value=0  inPortNames=[' '; ' '; ' '; ' '; ' '; ' '; ' '; ' '; ' '; ' '; ' '; ' '; ' '; ' '; ' '; ' '; ]  outPortNames=[' ']  dspbaimage=dspba_prim.jpg  text=fprintf('|');  style=Optimised  visibilities=8+2  version=20090407
  SampleDelay{,1..33} (34 alike) : DSPBAPrim/SampleDelay  primtype=sampdelay  nInputs=1  nOutputs=1  omode=Inherit via internal rule  otype=sfix(16)  scale=2^-15  rndmethod=Unbiased  factor=1  satmethod=Symmetric  shift_vec=[0 1 2 -1]  value=1  inPortNames=[' '; ' ';]  outPortNames=[' ']  dspbaimage=dspba_prim.jpg  text=dpoly(1, eye(1,value+1), 'z')  style=Optimised  visibilities=8 + 1024 + 2^17 + 2^18  flexible=off  slackgroup=0  augmented=0  version=20090407  advOptions=[]
  Scope : Scope  NumInputPorts=2
  SynthesisInfo : DSPBAPrim/SynthesisInfo  primtype=synthinfo  nInputs=0  nOutputs=0  omode=Inherit via internal rule  otype=sfix(16)  scale=2^-15  rndmethod=Truncate  factor=1  satmethod=Symmetric  shift_vec=[0 1 2 -1]  value=99  inPortNames=[' '; ' ';]  outPortNames=[' ']  dspbaimage=dspba_prim_ctrl.jpg  text=fprintf('Style=%s', style);  style=Scheduled  visibilities=2^15+2^17+2^18+2^19  constraintInUse=on  constraintRelation==  constraintLimit=7  bitAccurate=off  version=20150220
  single_delay12 : Subsystem  Commented=on
  vout : Outport
  cout : Outport  Port=2
  M0 : Outport  Port=3
  M1 : Outport  Port=4
  M2 : Outport  Port=5
  M3 : Outport  Port=6
  M4 : Outport  Port=7
  M5 : Outport  Port=8
  M6 : Outport  Port=9
  M7 : Outport  Port=10
  M8 : Outport  Port=11
  M9 : Outport  Port=12
  M10 : Outport  Port=13
  M11 : Outport  Port=14
  wires:
  Mux11/1 -> SampleDelay10/1
  Mux10/1 -> SampleDelay9/1
  Mux9/1 -> SampleDelay8/1
  Mux8/1 -> SampleDelay7/1
  Mux7/1 -> SampleDelay6/1
  Mux6/1 -> SampleDelay5/1
  Mux5/1 -> SampleDelay4/1
  Mux4/1 -> SampleDelay3/1
  Mux3/1 -> SampleDelay2/1
  Mux2/1 -> SampleDelay/1
  Mux1/1 -> SampleDelay1/1
  ChannelIn/3 -> MultAcc11/3, MultAcc10/3, MultAcc9/3, MultAcc8/3, MultAcc7/3, MultAcc6/3, MultAcc5/3, MultAcc4/3, MultAcc3/3, MultAcc2/3, MultAcc1/3, MultAcc/3  "q0"
  ChannelIn/4 -> Mux/3
  Or/1 -> Not/1
  valid/1 -> ChannelIn/1  "qv"
  channel/1 -> ChannelIn/2  "qc"
  Bi-Bq/1 -> ChannelIn/3  "q0"
  Ai/1 -> ChannelIn/4
  Acc_clear/1 -> ChannelIn/5
  ChannelOut/1 -> vout/1
  ChannelOut/2 -> cout/1
  ChannelOut/3 -> M0/1
  ChannelOut/4 -> M1/1
  ChannelOut/5 -> M2/1
  ChannelOut/6 -> M3/1
  ChannelOut/7 -> M4/1
  ChannelOut/8 -> M5/1
  ChannelOut/9 -> M6/1
  ChannelOut/10 -> M7/1
  ChannelOut/11 -> M8/1
  ChannelOut/12 -> M9/1
  ChannelOut/13 -> M10/1
  ChannelOut/14 -> M11/1
  MultAcc/1 -> ChannelOut/3
  MultAcc1/1 -> ChannelOut/4
  MultAcc2/1 -> ChannelOut/5
  MultAcc3/1 -> ChannelOut/6
  MultAcc4/1 -> ChannelOut/7
  MultAcc5/1 -> ChannelOut/8
  MultAcc6/1 -> ChannelOut/9
  MultAcc7/1 -> ChannelOut/10
  MultAcc8/1 -> ChannelOut/11
  MultAcc9/1 -> ChannelOut/12
  MultAcc10/1 -> ChannelOut/13
  MultAcc11/1 -> ChannelOut/14
  ChannelIn/2 -> ChannelOut/2  "qc"
  Const/1 -> Mux/2
  Const1/1 -> Mux1/2
  Const2/1 -> Mux2/2
  Const3/1 -> Mux3/2
  Const4/1 -> Mux4/2
  Const5/1 -> Mux5/2
  Const6/1 -> Mux6/2
  Const7/1 -> Mux7/2
  Const8/1 -> Mux8/2
  Const9/1 -> Mux9/2
  Const10/1 -> Mux10/2
  Const11/1 -> Mux11/2
  SampleDelay/1 -> Mux14/3, Mux3/3
  SampleDelay1/1 -> Mux12/3, Mux2/3
  SampleDelay2/1 -> Mux15/3, Mux4/3
  SampleDelay3/1 -> Mux16/3, Mux5/3
  SampleDelay4/1 -> Mux17/3, Mux6/3
  SampleDelay5/1 -> Mux18/3, Mux7/3
  SampleDelay6/1 -> Mux19/3, Mux8/3
  SampleDelay7/1 -> Mux20/3, Mux9/3
  SampleDelay8/1 -> Mux21/3, Mux10/3
  SampleDelay9/1 -> Mux22/3, Mux11/3
  SampleDelay10/1 -> Mux23/3
  ChannelIn/1 -> Scope/1, SampleDelay12/1, Mux/1  "qv"
  ChannelIn/5 -> Or/2
  SOP_in/1 -> ChannelIn/6
  ChannelIn/6 -> Or/1
  SampleDelay12/1 -> SampleDelay13/1, Mux1/1
  SampleDelay13/1 -> SampleDelay14/1, Mux2/1
  SampleDelay14/1 -> SampleDelay15/1, Mux3/1
  SampleDelay15/1 -> SampleDelay16/1, Mux4/1
  SampleDelay16/1 -> SampleDelay17/1, Mux5/1
  SampleDelay17/1 -> SampleDelay18/1, Mux6/1
  SampleDelay18/1 -> SampleDelay19/1, Mux7/1
  SampleDelay19/1 -> SampleDelay20/1, Mux8/1
  SampleDelay20/1 -> SampleDelay21/1, Mux9/1
  SampleDelay21/1 -> SampleDelay22/1, Mux10/1
  SampleDelay22/1 -> ChannelOut/1, Mux11/1
  SampleDelay23/1 -> Mux12/1, MultAcc1/1, SampleDelay24/1
  SampleDelay24/1 -> MultAcc2/1, Mux14/1, SampleDelay25/1
  SampleDelay25/1 -> MultAcc3/1, Mux15/1, SampleDelay26/1
  SampleDelay26/1 -> MultAcc4/1, Mux16/1, SampleDelay27/1
  SampleDelay27/1 -> MultAcc5/1, Mux17/1, SampleDelay28/1
  SampleDelay28/1 -> MultAcc6/1, Mux18/1, SampleDelay29/1
  SampleDelay29/1 -> MultAcc7/1, Mux19/1, SampleDelay30/1
  SampleDelay30/1 -> Mux20/1, MultAcc8/1, SampleDelay31/1
  SampleDelay31/1 -> MultAcc9/1, Mux21/1, SampleDelay32/1
  SampleDelay32/1 -> Mux22/1, MultAcc10/1, SampleDelay33/1
  SampleDelay33/1 -> MultAcc11/1, Mux23/1
  Mux/1 -> SampleDelay11/1
  SampleDelay11/1 -> Mux13/3, Mux1/3
  Not/1 -> MultAcc/1, Mux13/1, Scope/2, SampleDelay23/1
  Const13/1 -> Mux13/2
  Mux13/1 -> MultAcc/2
  Const12/1 -> Mux12/2
  Mux12/1 -> MultAcc1/2
  Const14/1 -> Mux14/2
  Mux14/1 -> MultAcc2/2
  Const15/1 -> Mux15/2
  Mux15/1 -> MultAcc3/2
  Const16/1 -> Mux16/2
  Mux16/1 -> MultAcc4/2
  Const17/1 -> Mux17/2
  Mux17/1 -> MultAcc5/2
  Const18/1 -> Mux18/2
  Mux18/1 -> MultAcc6/2
  Const19/1 -> Mux19/2
  Mux19/1 -> MultAcc7/2
  Const20/1 -> Mux20/2
  Mux20/1 -> MultAcc8/2
  Const21/1 -> Mux21/2
  Mux21/1 -> MultAcc9/2
  Const22/1 -> Mux22/2
  Mux22/1 -> MultAcc10/2
  Const23/1 -> Mux23/2
  Mux23/1 -> MultAcc11/2
